simulink model "BuzzerWithLights"  (R2021b)
settings: Solver=FixedStepAuto  StartTime=0.0  StopTime=20  RelTol=1e-3  EnableMultiTasking=on
libraries: explorerHatPro x3, raspberrypiBasiclib x1
settings Model: Creator=ebene  LastModifiedBy=ebene
settings SolverCC: PositivePriorityOrder=on
settings DataIOCC: ReturnWorkspaceOutputs=off
settings OptimizationCC: EnhancedBackFolding=on  PassReuseOutputArgsAs=Individual arguments  ZeroExternalMemoryAtStartup=off  ZeroInternalMemoryAtStartup=off  MaxStackSize=64  OptimizeBlockOrder=speed  DifferentSizesBufferReuse=on  OptimizationCustomize=off  EfficientTunableParamExpr=on
settings DebuggingCC: ParameterTunabilityLossMsg=error
settings HardwareCC: ProdBitPerPointer=32  ProdBitPerSizeT=32  ProdBitPerPtrDiffT=32  ProdLargestAtomicInteger=Long  ProdLargestAtomicFloat=Double  ProdWordSize=32  ProdLongLongMode=on  ProdHWDeviceType=ARM Compatible->ARM Cortex  UseEmbeddedCoderFeatures=off
settings RTWCC: Description=Embedded Coder  SystemTargetFile=ert.tlc  HardwareBoard=Raspberry Pi  TLCOptions="-aInlineSetEventsForThisBaseRateFcn=TLC_FALSE -aSuppressMultiTaskScheduler=TLC_FALSE  -aRateBasedStepFcn=0"  TemplateMakefile=ert_default_tmf  Toolchain=GNU GCC Embedded Linux  BuildConfiguration=Faster Runs
settings CodeAppCC: ForceParamTrailComments=on  OperatorAnnotations=on  SimulinkDataObjDesc=on  SFDataObjDesc=on  InsertBlockDesc=on
settings ERTTargetCC: SupportNonInlinedSFcns=on  SupportVariableSizeSignals=on  ExtMode=on  ExtModeTransport=2  ExtModeStaticAlloc=on  ExtModeMexFile=ext_xcp  ExtModeMexArgs='192.168.1.106' 0 17725  ExtModeIntrfLevel=Level2 - Open  ERTSrcFileBannerTemplate=codertarget_code_template.cgt  ERTHdrFileBannerTemplate=codertarget_code_template.cgt  ERTDataSrcFileTemplate=codertarget_code_template.cgt  ERTDataHdrFileTemplate=codertarget_code_template.cgt

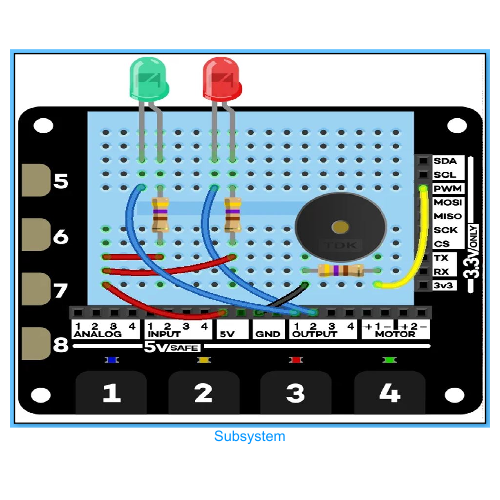
[thumbnail: Simulink's stored preview of the top-level diagram]
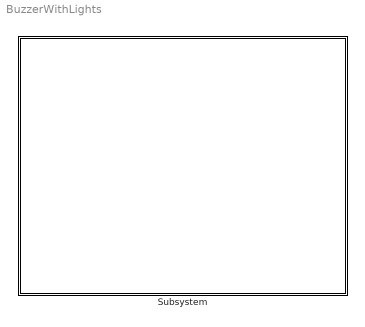
== system BuzzerWithLights ==
  Subsystem : Subsystem
      mask Display: image(imread('src/ExplorerHat/icons/buzzer.jpg'))

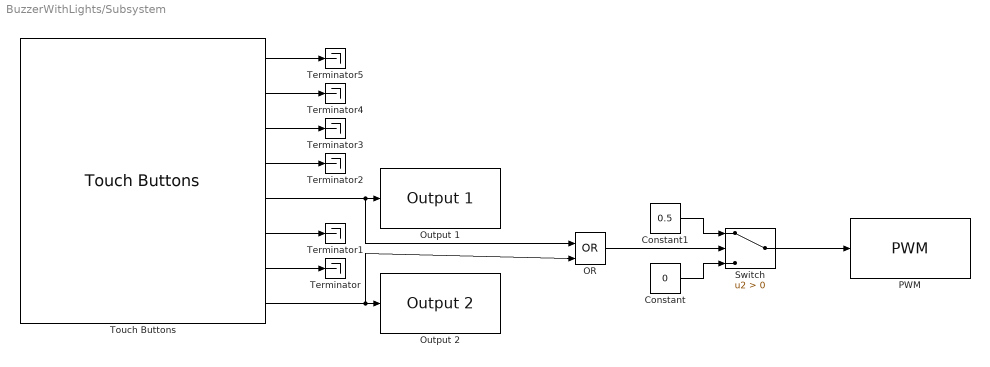
== system BuzzerWithLights/Subsystem ==
  Constant : Constant  Value=0
  Constant1 : Constant  Value=0.5
  OR : Logic  Operator=OR  IconShape=distinctive  AllPortsSameDT=off
  Output 1 : explorerHatPro/Output 1  SystemSampleTime=-1  VariantActivationTime=update diagram  Latency=0  AutoFrameSizeCalculation=off
      settings: SourceProductName=Explorer Hat Pro
  Output 2 : explorerHatPro/Output 2  SystemSampleTime=-1  VariantActivationTime=update diagram  Latency=0  AutoFrameSizeCalculation=off
      settings: SourceProductName=Explorer Hat Pro
  PWM : raspberrypiBasiclib/PWM  board=Pi 4 Model B  Pin_=18  Frequency=400  blockPlatform=Raspberry Pi
      settings: SourceProductBaseCode=RASPPI
  Switch : Switch  Criteria=u2 > Threshold
  Terminator{,1..5} (6 alike) : Terminator
  Touch Buttons : explorerHatPro/Touch Buttons  SampleTime=0.01
      settings: SourceProductName=Explorer Hat Pro
  wires:
  Touch Buttons/2 -> Terminator4/1
  Touch Buttons/6 -> Terminator1/1
  Touch Buttons/8 -> OR/2, Output 2/1
  Touch Buttons/3 -> Terminator3/1
  Touch Buttons/1 -> Terminator5/1
  Switch/1 -> PWM/1
  Constant1/1 -> Switch/1
  Touch Buttons/5 -> OR/1, Output 1/1
  Touch Buttons/4 -> Terminator2/1
  Touch Buttons/7 -> Terminator/1
  OR/1 -> Switch/2
  Constant/1 -> Switch/3
